simulink model "heater"  (Simulink 7.8)
settings: Solver=ode45  StartTime=0.0  StopTime=400  RelTol=1e-3
values from neighbouring files (symbols this model uses):
  K_D = 3*K_u*T_u/40    (= 2.764125)    [parameters.m]
  K_I = 1.2*K_u/T_u    (= 0.00323076923077)    [parameters.m]
  K_P = 0.6*K_u    (= 0.189)    [parameters.m]
libraries: simulink x3
settings Model: Creator=joob  LastModifiedBy=joob

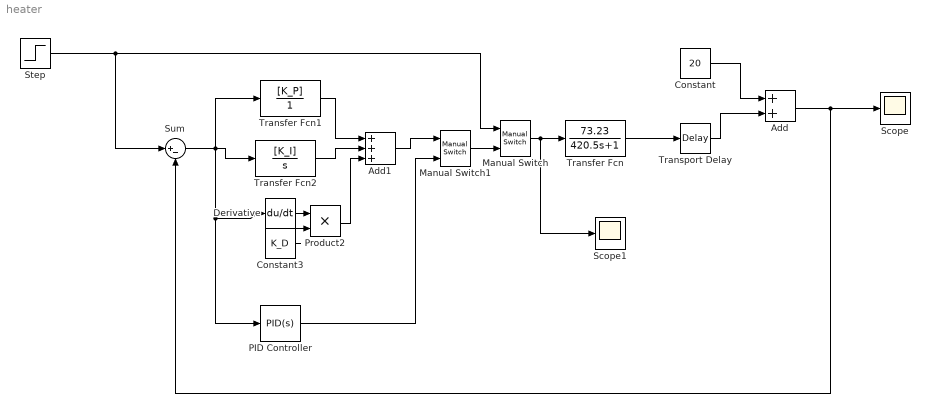
== system heater ==
  Add : Sum
  Add1 : Sum  Inputs=+++
  Constant : Constant  Value=20
  Constant3 : Constant  Value=K_D
  Derivative : Derivative
  Manual Switch : simulink/Signal Routing/Manual Switch  sw=0  action=0  varsize=off
  Manual Switch1 : simulink/Signal Routing/Manual Switch  sw=1  action=0  varsize=off
  PID Controller : simulink/Continuous/PID Controller  Controller=PID  TimeDomain=Continuous-time  SampleTime=1  IntegratorMethod=Forward Euler  FilterMethod=Forward Euler  Form=Parallel  P=K_P  I=K_I  D=K_D  N=100  InitialConditionSource=internal  InitialConditionForIntegrator=0  InitialConditionForFilter=0  ExternalReset=none  LimitOutput=off  UpperSaturationLimit=inf  LowerSaturationLimit=-inf  LinearizeAsGain=off  AntiWindupMode=none  Kb=1  TrackingMode=off  Kt=1  PParamMin=[]  PParamMax=[]  IParamMin=[]  IParamMax=[]  DParamMin=[]  DParamMax=[]  NParamMin=[]  NParamMax=[]  KbParamMin=[]  KbParamMax=[]  KtParamMin=[]  KtParamMax=[]  POutMin=[]  POutMax=[]  IOutMin=[]  IOutMax=[]  DOutMin=[]  DOutMax=[]  NOutMin=[]  NOutMax=[]  KbOutMin=[]  KbOutMax=[]  KtOutMin=[]  KtOutMax=[]  IntegratorOutMin=[]  IntegratorOutMax=[]  FilterOutMin=[]  FilterOutMax=[]  SumOutMin=[]  SumOutMax=[]  SumI1OutMin=[]  SumI1OutMax=[]  SumI2OutMin=[]  SumI2OutMax=[]  SumI3OutMin=[]  SumI3OutMax=[]  SumDOutMin=[]  SumDOutMax=[]  SaturationOutMin=[]  SaturationOutMax=[]  IntegratorContinuousStateAttributes=''  IntegratorStateMustResolveToSignalObject=off  IntegratorRTWStateStorageClass=Auto  FilterContinuousStateAttributes=''  FilterStateMustResolveToSignalObject=off  FilterRTWStateStorageClass=Auto
  Product2 : Product  RndMeth=Zero
  Scope : Scope
  Scope1 : Scope
  Step : Step  Time=0  After=25  SampleTime=0
  Sum : Sum  Inputs=|+-
  Transfer Fcn : TransferFcn  Numerator=[73.23]  Denominator=[420.5 1]
  Transfer Fcn1 : TransferFcn  Numerator=[K_P]  Denominator=[1]
  Transfer Fcn2 : TransferFcn  Numerator=[K_I]  Denominator=[1 0]
  Transport Delay : TransportDelay  DelayTime=30
  wires:
  Constant/1 -> Add/1
  Transfer Fcn/1 -> Transport Delay/1
  Transport Delay/1 -> Add/2
  Manual Switch/1 -> Transfer Fcn/1, Scope1/1
  Add/1 -> Sum/2, Scope/1
  Step/1 -> Manual Switch/1, Sum/1
  Transfer Fcn1/1 -> Add1/1
  Transfer Fcn2/1 -> Add1/2
  Product2/1 -> Add1/3
  Sum/1 -> Transfer Fcn2/1, Transfer Fcn1/1, Derivative/1, PID Controller/1
  Constant3/1 -> Product2/2
  Derivative/1 -> Product2/1
  Manual Switch1/1 -> Manual Switch/2
  Add1/1 -> Manual Switch1/1
  PID Controller/1 -> Manual Switch1/2
